simulink model "HIL_comm"  (R2022a)
settings: Solver=FixedStepAuto  StartTime=0.0  StopTime=10.0  FixedStep=control_TimeStep  RelTol=1e-3
undefined symbols (not defined in the file): param, param_vdc, vdc_TimeStep
libraries: instrumentseriallib x3, slrealtimeutilitieslib x2
settings Model: Creator=Usuario  LastModifiedBy=Usuario

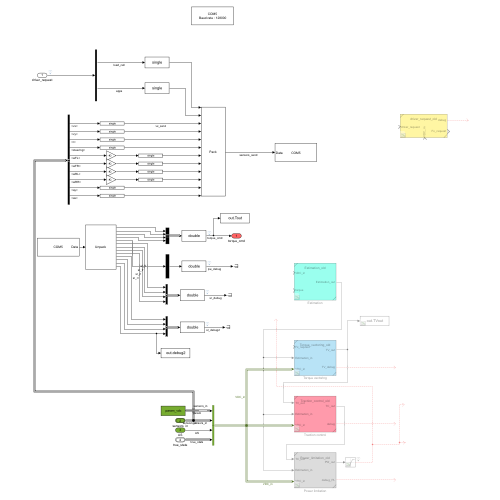
[thumbnail: Simulink's stored preview of the top-level diagram]
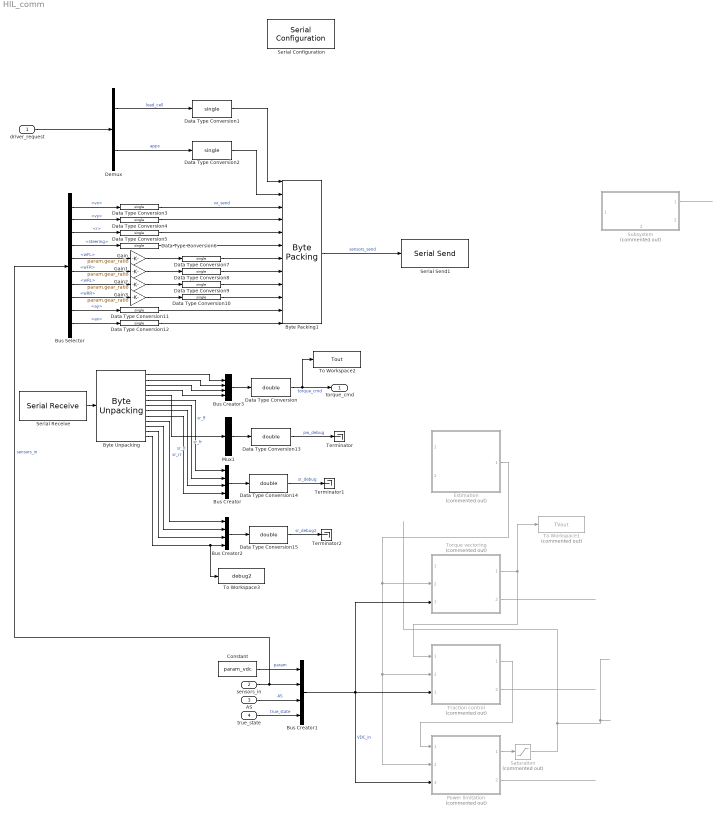
== system HIL_comm ==
  driver_request : Inport
  sensors_in : Inport  Port=2  OutDataTypeStr=Bus: sensorBus
  AS : Inport  Port=3
  true_state : Inport  Port=4  OutDataTypeStr=Bus: stateBus
  Bus Creator{,1..3} (4 alike) : BusCreator  Inputs=4
  Bus Selector : BusSelector  OutputSignals=gss.vx,gss.vy,gss.r,ext.steering,encoder.wFL,encoder.wFR,encoder.wRL,encoder.wRR,IMU.ay,IMU.ax
  Byte Packing1 : slrealtimeutilitieslib/Byte Packing  MaskPackedDataType=uint8  MaskUnpackedDataTypes={'single','single','single','single','single','single','single','single','single','single','single','single'}  MaskAlignment=1
  Byte Unpacking : slrealtimeutilitieslib/Byte Unpacking  MaskUnpackedDataTypes={'single','single','single','single','single','single','single','single','single','single','single','single','single'}  MaskUnpackedDataSizes={[1],[1],[1],[1],[1],[1],[1],[1],[1],[1],[1],[1],[1]}  MaskAlignment=1
      settings: SourceProductBaseCode=XP
  Constant : Constant  Value=param_vdc  OutDataTypeStr=Bus: vdcBus
  Data Type Conversion{,13..15} (4 alike) : DataTypeConversion  OutDataTypeStr=double  SaturateOnIntegerOverflow=off  RndMeth=Floor
  Data Type Conversion{1..12} (12 alike) : DataTypeConversion  OutDataTypeStr=single  SaturateOnIntegerOverflow=off  RndMeth=Floor
  Demux : Demux  Outputs=2
  Estimation : Subsystem  Commented=on  ReferencedSubsystem=Estimation_old
  Gain{,1..3} (4 alike) : Gain  Gain=param.gear_ratio
  Mux1 : Mux  Inputs=1
  Power limitation : Subsystem  Commented=on  ReferencedSubsystem=Power_limitation_old
  Saturation : Saturate  Commented=on  UpperLimit=param.torque_limit_positive  LowerLimit=param.torque_limit_negative
  Serial Configuration : instrumentseriallib/Serial Configuration  Priority=-200000  PortSel=COM5  Port=COM5  ComPort=COM5  BaudRate=128000  DataBits=8  Parity=none  StopBits=1  ByteOrder=little-endian  FlowControl=none  Timeout=10  SimulateUsing=Interpreted execution  BlockInModel=on  aMode=1
      settings: SourceProductBaseCode=OT,IC,MT
  Serial Receive : instrumentseriallib/Serial Receive  Priority=1  PortSel=COM5  Port=COM5  ComPort=COM5  DataType=uint8  SaveDataType=uint8  ToggleHeader=on  Header=[171 205 2]  ToggleTerminator=off  Terminator=<none>  CustomTerminator=[]  InputFormat=Column major  ToggleDataSize=on  DataSize=[52 1]  EnableBlockingMode=on  ActionDataUnavailable=Output last received value  ActionWhenDataUnavailable=Output last received value  CustomValue=0  SampleTime=vdc_TimeStep  SimulateUsing=Interpreted execution  BlockInModel=on  aMode=1
      settings: SourceProductBaseCode=OT,IC,MT
  Serial Send1 : instrumentseriallib/Serial Send  Priority=1  PortSel=COM5  Port=COM5  ComPort=COM5  Header=[171 205 1]  Terminator=<none>  CustomTerminator=[]  EnableBlockingMode=off  SimulateUsing=Interpreted execution  BlockInModel=on  aMode=1
      settings: SourceProductBaseCode=OT,IC,MT
  Subsystem : Subsystem  Commented=on  ReferencedSubsystem=driver_request_old
      settings: PortSchema="{\"entries\":[{\"content\":{\"sides\":[{\"content\":{\"connectorIds\":[\"In1\"]},\"type\":\"ConnectorPlacement.EquallySpacedRectSide\",\"uuid\":\"6d0b78b3-ffc0-496d-8d3a-7ba3f556f803\"},{\"content\":{\"connectorIds\":[\"Out1\",\"Out2\"],\"side\":\"RIGHT\"},\"type\":\"ConnectorPlacement.EquallySpacedRectSide\",\"uuid\":\"be1dfba9-3592-437e-9363-a3609142bbc4\"},{\"content\":{\"connectorIds\":[],\"side\":\"TOP\"},\"type\":\"ConnectorPlacement.EquallySpacedRectSide\",\"uuid\":\"ddffd853-c46f-4213-b654-9451d95e6853\"},{\"content\":{\"connectorIds\":[\"In2\"],\"side\":\"BOTTOM\"},\"type\":\"ConnectorPlacement.EquallySpacedRectSide\",\"uuid\":\"b463dc20-ae30-4837-a1c3-1d0c4501f548\"}]},\"type\":\"ConnectorPlacement.EquallySpacedConnector\",\"uuid\":\"75a8dd9f-93ed-4a7a-b725-fd6938405663\"}],\"packageUris\":[\"http://schema.mathworks.com/mf0/Connector/R2020b\"],\"version\":\"1.0\"}"
  Terminator : Terminator
  Terminator1 : Terminator
  Terminator2 : Terminator
  To Workspace1 : ToWorkspace  Commented=on  VariableName=TVout  SaveFormat=Timeseries  SampleTime=-1
  To Workspace2 : ToWorkspace  VariableName=Tout  SaveFormat=Structure With Time  SampleTime=-1
  To Workspace3 : ToWorkspace  VariableName=debug2  SaveFormat=Structure With Time  SampleTime=-1
  Torque vectoring : Subsystem  Commented=on  ReferencedSubsystem=Torque_vectoring_old
  Traction control : Subsystem  Commented=on  ReferencedSubsystem=Traction_control_old
  torque_cmd : Outport
  wires:
  Data Type Conversion/1 -> torque_cmd/1, To Workspace2/1  "torque_cmd"
  Data Type Conversion1/1 -> Byte Packing1/1
  Bus Creator3/1 -> Data Type Conversion/1
  Byte Unpacking/1 -> Bus Creator3/1
  Serial Receive/1 -> Byte Unpacking/1
  Torque vectoring/2 -> ?
  Saturation/1 -> ?
  Estimation/1 -> Torque vectoring/2, Traction control/2, Power limitation/2
  true_state/1 -> Bus Creator1/4  "true_state"
  Traction control/1 -> Power limitation/1
  Power limitation/2 -> ?
  sensors_in/1 -> Bus Selector/1, Bus Creator1/2  "sensors_in"
  AS/1 -> Bus Creator1/3  "AS"
  Subsystem/1 -> ?
  Torque vectoring/1 -> To Workspace1/1, Traction control/1
  Bus Creator1/1 -> Torque vectoring/3, Power limitation/3, Traction control/3  "VDC_in"
  Power limitation/1 -> Saturation/1
  Constant/1 -> Bus Creator1/1  "param"
  Traction control/2 -> ?
  driver_request/1 -> Demux/1
  Demux/1 -> Data Type Conversion1/1  "load_cell"
  Data Type Conversion2/1 -> Byte Packing1/2
  Demux/2 -> Data Type Conversion2/1  "apps"
  Bus Selector/1 -> Data Type Conversion3/1  "<vx>"
  Bus Selector/2 -> Data Type Conversion4/1  "<vy>"
  Bus Selector/3 -> Data Type Conversion5/1  "<r>"
  Bus Selector/10 -> Data Type Conversion12/1  "<ax>"
  Bus Selector/9 -> Data Type Conversion11/1  "<ay>"
  Bus Selector/8 -> Gain3/1  "<wRR>"
  Bus Selector/7 -> Gain2/1  "<wRL>"
  Bus Selector/6 -> Gain1/1  "<wFR>"
  Bus Selector/5 -> Gain/1  "<wFL>"
  Bus Selector/4 -> Data Type Conversion6/1  "<steering>"
  Byte Packing1/1 -> Serial Send1/1  "sensors_send"
  Data Type Conversion3/1 -> Byte Packing1/3  "vx_send"
  Data Type Conversion4/1 -> Byte Packing1/4
  Data Type Conversion5/1 -> Byte Packing1/5
  Data Type Conversion6/1 -> Byte Packing1/6
  Data Type Conversion7/1 -> Byte Packing1/7
  Data Type Conversion8/1 -> Byte Packing1/8
  Data Type Conversion9/1 -> Byte Packing1/9
  Data Type Conversion10/1 -> Byte Packing1/10
  Data Type Conversion11/1 -> Byte Packing1/11
  Data Type Conversion12/1 -> Byte Packing1/12
  Byte Unpacking/2 -> Bus Creator3/2
  Byte Unpacking/3 -> Bus Creator3/3
  Byte Unpacking/4 -> Bus Creator3/4
  Byte Unpacking/5 -> Mux1/1
  Mux1/1 -> Data Type Conversion13/1
  Data Type Conversion13/1 -> Terminator/1  "pw_debug"
  Gain/1 -> Data Type Conversion7/1
  Gain1/1 -> Data Type Conversion8/1
  Gain2/1 -> Data Type Conversion9/1
  Gain3/1 -> Data Type Conversion10/1
  Byte Unpacking/9 -> Bus Creator/4  "sr_rr"
  Byte Unpacking/8 -> Bus Creator/3  "sr_rl"
  Byte Unpacking/7 -> Bus Creator/2  "sr_fr"
  Byte Unpacking/6 -> Bus Creator/1  "sr_fl"
  Bus Creator/1 -> Data Type Conversion14/1
  Data Type Conversion14/1 -> Terminator1/1  "sr_debug"
  Byte Unpacking/13 -> To Workspace3/1, Bus Creator2/4
  Byte Unpacking/12 -> Bus Creator2/3
  Byte Unpacking/11 -> Bus Creator2/2
  Byte Unpacking/10 -> Bus Creator2/1
  Bus Creator2/1 -> Data Type Conversion15/1
  Data Type Conversion15/1 -> Terminator2/1  "sr_debug2"
